simulink model "dc_motor_control"  (R2018b)
settings: Solver=ode1  StartTime=0.0  StopTime=3  FixedStep=1E-6  RelTol=1e-3
model workspace (MAT data in the model file):
  B = 0
  J = 7.66e-09
  K = 0.00205
  L = 7.26e-05
  R = 4.07
libraries: simulink x1
settings Model: OrderedModelArguments=off  Creator=takuya  LastModifiedBy=takuya
settings DataIOCC: ReturnWorkspaceOutputs=on

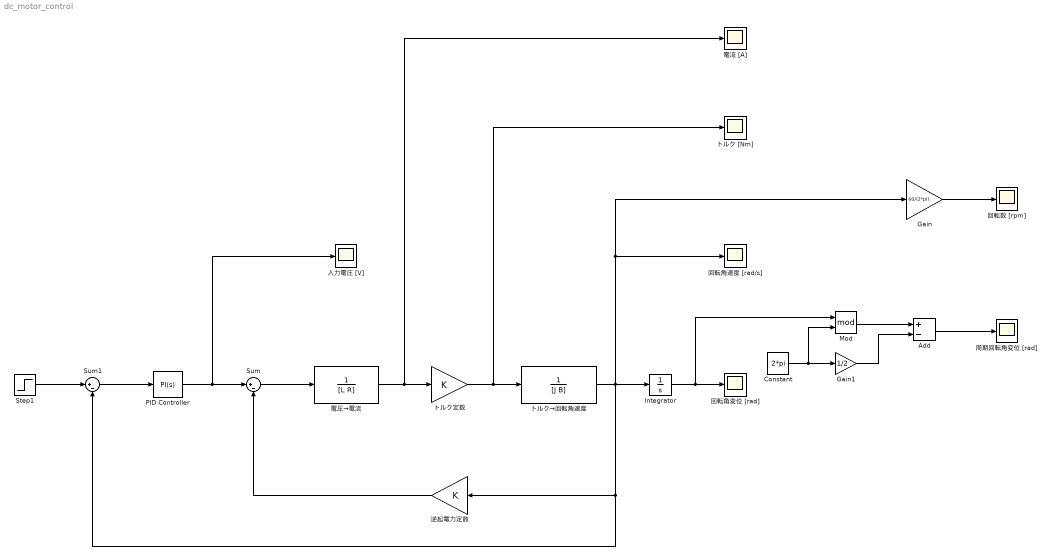
== system dc_motor_control ==
  Add : Sum  Inputs=+-
  Constant : Constant  Value=2*pi
  Gain : Gain  Gain=60/(2*pi)
  Gain1 : Gain  Gain=1/2
  Integrator : Integrator
  Mod : Math  Operator=mod  SaturateOnIntegerOverflow=on
  PID Controller : simulink/Continuous/PID Controller  Controller=PI  Form=Parallel  TimeDomain=Continuous-time  SampleTime=-1  IntegratorMethod=Forward Euler  FilterMethod=Forward Euler  ControllerParametersSource=internal  P=0.001  I=0.01  D=0  UseFilter=on  N=100  TunerSelectOption=Transfer Function Based (PID Tuner App)  InitialConditionSource=internal  InitialConditionForIntegrator=0  InitialConditionForFilter=0  DifferentiatorICPrevScaledInput=0  ExternalReset=none  TrackingMode=off  Kt=1  LimitOutput=off  UpperSaturationLimit=inf  LowerSaturationLimit=-inf  LinearizeAsGain=on  AntiWindupMode=none  Kb=1  POutMin=[]  POutMax=[]  IOutMin=[]  IOutMax=[]  DOutMin=[]  DOutMax=[]  NOutMin=[]  NOutMax=[]  SumOutMin=[]  SumOutMax=[]  SaturationOutMin=[]  SaturationOutMax=[]  PParamMin=[]  PParamMax=[]  IParamMin=[]  IParamMax=[]  DParamMin=[]  DParamMax=[]  NParamMin=[]  NParamMax=[]  KbParamMin=[]  KbParamMax=[]  KtParamMin=[]  KtParamMax=[]  KbOutMin=[]  KbOutMax=[]  KtOutMin=[]  KtOutMax=[]  IntegratorOutMin=[]  IntegratorOutMax=[]  FilterOutMin=[]  FilterOutMax=[]  SumI1OutMin=[]  SumI1OutMax=[]  SumI2OutMin=[]  SumI2OutMax=[]  SumI3OutMin=[]  SumI3OutMax=[]  SumI4OutMin=[]  SumI4OutMax=[]  SumDOutMin=[]  SumDOutMax=[]  DifferentiatorOutMin=[]  DifferentiatorOutMax=[]  FilterDiffOutCoefMin=[]  FilterDiffOutCoefMax=[]  ReciprocalOutMin=[]  ReciprocalOutMax=[]  SumDenOutMin=[]  SumDenOutMax=[]  SumNumOutMin=[]  SumNumOutMax=[]  DivideOutMin=[]  DivideOutMax=[]  IntegratorContinuousStateAttributes=''  IntegratorStateMustResolveToSignalObject=off  IntegratorRTWStateStorageClass=Auto  FilterContinuousStateAttributes=''  FilterStateMustResolveToSignalObject=off  FilterRTWStateStorageClass=Auto  ParallelPVariant=InternalParameters  IdealPVariant=Disabled  IVariant=InternalParameters  DVariant=Disabled  IntegratorVariant=Continuous  SatVariant=Disabled  AWVariant=Passthrough  PCopyVariant=Disabled  TRVariant=Disabled  FdbkBlocksVariant=Forward  IdealPFdbkVariant=Disabled  SatFdbkVariant=Disabled  DerivativeFilterVariant=Disabled  NVariant=Disabled  NCopyVariant=Disabled_SignalSpec  FilterICVariant=Disabled  IntegratorICVariant=InternalICs  ExternalResetVariant=Disabled  TRSumVariant=Passthrough  SumFdbkVariant=Disabled  SumVariant=Sum_PI
  Step1 : Step  Time=0  After=(2 * pi / 60) * 500  SampleTime=0
  Sum : Sum  Inputs=|+-
  Sum1 : Sum  Inputs=|+-
  トルク [Nm] : Scope
  トルク→回転角速度 : TransferFcn  Denominator=[J B]
  トルク定数 : Gain  Gain=K
  入力電圧 [V] : Scope
  周期回転角変位 [rad] : Scope
  回転数 [rpm] : Scope
  回転角変位 [rad] : Scope
  回転角速度 [rad/s] : Scope
  逆起電力定数 : Gain  Gain=K
  電圧→電流 : TransferFcn  Denominator=[L R]
  電流 [A] : Scope
  wires:
  逆起電力定数/1 -> Sum/2
  Integrator/1 -> Mod/1, 回転角変位 [rad]/1
  Gain/1 -> 回転数 [rpm]/1
  Constant/1 -> Mod/2, Gain1/1
  Mod/1 -> Add/1
  Gain1/1 -> Add/2
  Add/1 -> 周期回転角変位 [rad]/1
  電圧→電流/1 -> 電流 [A]/1, トルク定数/1
  トルク→回転角速度/1 -> Gain/1, 回転角速度 [rad/s]/1, 逆起電力定数/1, Sum1/2, Integrator/1
  Sum/1 -> 電圧→電流/1
  PID Controller/1 -> 入力電圧 [V]/1, Sum/1
  Sum1/1 -> PID Controller/1
  Step1/1 -> Sum1/1
  トルク定数/1 -> トルク [Nm]/1, トルク→回転角速度/1
